simulink model "ejemplo3"  (R2018a)
settings: Solver=VariableStepAuto  StartTime=0.0  StopTime=10.0  RelTol=1e-3
InitFcn:
  | ejemplo_2
values from neighbouring files (symbols this model uses):
  ki = kt(1,3)    [control_nolineal_linealizacion_entrada_estado.m]    (also in e_mimo.m; ej_mimo.m = kt(:,2+1:end); ej_mimo2.m = kt(:,2+1:end); ejemplo_2.m)
  kp = kt(1,1:2)    [control_nolineal_linealizacion_entrada_estado.m]    (also in e_mimo.m; ej_mimo.m = kt(:,1:2); ej_mimo2.m = kt(:,1:2); ejemplo_2.m)
libraries: simulink x1
settings Model: Creator=carma  LastModifiedBy=carma

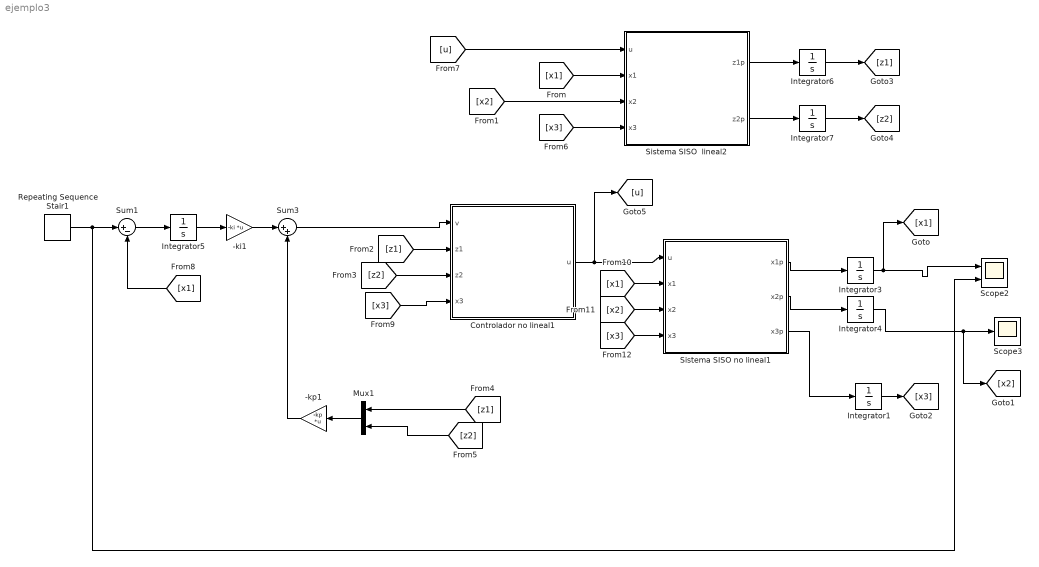
== system ejemplo3 ==
  -ki1 : Gain  Gain=-ki  Multiplication=Matrix(K*u) (u vector)
  -kp1 : Gain  Gain=-kp  Multiplication=Matrix(K*u) (u vector)
  Controlador no lineal1 : MATLAB Function  TreatAsAtomicUnit=on
  Integrator{1,3..7} (6 alike) : Integrator
  Mux1 : Mux  Inputs=2
  Repeating Sequence Stair1 : simulink/Sources/Repeating Sequence Stair  OutValues=[0.5 0.4 -0.2 0.1 0.3].'  tsamp=2  OutMin=[]  OutMax=[]  OutDataTypeStr=double  OutputDataTypeScalingMode=double  OutDataType=fixdt(0,8)  ConRadixGroup=Best Precision: Vector-wise  OutScaling=2^-12
  Scope2 : Scope  NumInputPorts=2
  Scope3 : Scope
  Sistema SISO  lineal2 : MATLAB Function  TreatAsAtomicUnit=on
  Sistema SISO no lineal1 : MATLAB Function  TreatAsAtomicUnit=on
  Sum1 : Sum  Inputs=|+-
  Sum3 : Sum  Inputs=|++
  wires:
  Repeating Sequence Stair1/1 -> Scope2/2, Sum1/1
  Sum3/1 -> Controlador no lineal1/1(v)
  Integrator3/1 -> [x1], Scope2/1
  Sistema SISO no lineal1/2(x2p) -> Integrator4/1
  Sum1/1 -> Integrator5/1
  Controlador no lineal1/1(u) -> [u], Sistema SISO no lineal1/1(u)
  Sistema SISO no lineal1/1(x1p) -> Integrator3/1
  Integrator4/1 -> [x2], Scope3/1
  Mux1/1 -> -kp1/1
  Integrator5/1 -> -ki1/1
  -ki1/1 -> Sum3/1
  -kp1/1 -> Sum3/2
  Sistema SISO no lineal1/3(x3p) -> Integrator1/1
  Integrator1/1 -> [x3]
  Integrator6/1 -> [z1]
  [x1] -> Sistema SISO  lineal2/2(x1)
  [x2] -> Sistema SISO  lineal2/3(x2)
  Integrator7/1 -> [z2]
  Sistema SISO  lineal2/1(z1p) -> Integrator6/1
  Sistema SISO  lineal2/2(z2p) -> Integrator7/1
  [z1] -> Controlador no lineal1/2(z1)
  [z2] -> Controlador no lineal1/3(z2)
  [z1] -> Mux1/1
  [z2] -> Mux1/2
  [x3] -> Sistema SISO  lineal2/4(x3)
  [u] -> Sistema SISO  lineal2/1(u)
  [x1] -> Sum1/2
  [x3] -> Controlador no lineal1/4(x3)
  [x1] -> Sistema SISO no lineal1/2(x1)
  [x2] -> Sistema SISO no lineal1/3(x2)
  [x3] -> Sistema SISO no lineal1/4(x3)

== matlab function ejemplo3/Controlador no lineal1 ==
  data: v input; u output; z1 input; z2 input; x3 input
function u = fcn(v,z1,z2,x3)

%parametros
a=4;


u=-3*z1^2*z2-z1^2+v-x3;

%s=5;
%syms y
%Cx3=(2+10^(pk2-y))/(1+10^(pk2-y)+10^(pk1+pk2-2*y));
%h=-x1+x2-x3*Cx3+10^(-y)-10^(y-pkw)==0;

%s=double(solve(h));

== matlab function ejemplo3/Sistema SISO no lineal1 ==
  data: u input; x1p output; x1 input; x2 input; x2p output; x3 input; x3p output
function [x1p,x2p,x3p]= fcn(u,x1,x2,x3)

%parametros
a=4;



x1p=x2+x1^3
x2p=x1^2+u+x3;
x3p=x1^2+u;

%s=5;
%syms y
%Cx3=(2+10^(pk2-y))/(1+10^(pk2-y)+10^(pk1+pk2-2*y));
%h=-x1+x2-x3*Cx3+10^(-y)-10^(y-pkw)==0;

%s=double(solve(h));

== matlab function ejemplo3/Sistema SISO  lineal2 ==
  data: u input; z1p output; x1 input; x2 input; z2p output; x3 input
function [z1p,z2p]= fcn(u,x1,x2,x3)

z1p=x2+x1^3;
z2p=u+x1^2+3*x1^2*(x2+x1^3)+x3;


% z1p=z2;
% z2p=v;

%s=5;
%syms y
%Cx3=(2+10^(pk2-y))/(1+10^(pk2-y)+10^(pk1+pk2-2*y));
%h=-x1+x2-x3*Cx3+10^(-y)-10^(y-pkw)==0;

%s=double(solve(h));
